simulink model "Sensors_Integrated"  (R2021b)
settings: Solver=FixedStepAuto  StartTime=0.0  StopTime=10.0  RelTol=1e-3
settings Model: Creator=Mohand  LastModifiedBy=Mohand
settings OptimizationCC: PassReuseOutputArgsAs=Individual arguments  OptimizeDataStoreBuffers=off  BusAssignmentInplaceUpdate=off  OptimizationLevel=level0  EfficientTunableParamExpr=on
settings DebuggingCC: ParameterTunabilityLossMsg=error
settings HardwareCC: ProdBitPerPointer=32  ProdBitPerSizeT=32  ProdBitPerPtrDiffT=32  ProdLargestAtomicInteger=Long  ProdLargestAtomicFloat=Double  ProdWordSize=32  ProdHWDeviceType=ARM Compatible->ARM Cortex-M
settings SFSimCC: MATLABDynamicMemAlloc=off
settings RTWCC: Description=Embedded Coder  SystemTargetFile=ert.tlc  GenCodeOnly=on  TemplateMakefile=ert_default_tmf  GenerateReport=on
settings CodeAppCC: ForceParamTrailComments=on  IgnoreCustomStorageClasses=off  OperatorAnnotations=on  SimulinkDataObjDesc=on  SFDataObjDesc=on  CustomSymbolStrGlobalVar=rt$N$M  CustomSymbolStrType=$N$M  CustomSymbolStrFcn=$N$M$F  InsertBlockDesc=on
settings ERTTargetCC: GenerateSampleERTMain=on  CodeInterfacePackaging=Reusable function  SupportComplex=off  SupportContinuousTime=on  ERTCustomFileTemplate=example_file_process.tlc

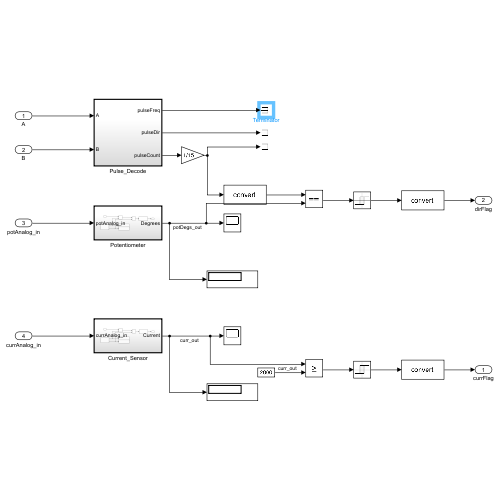
[thumbnail: Simulink's stored preview of the top-level diagram]
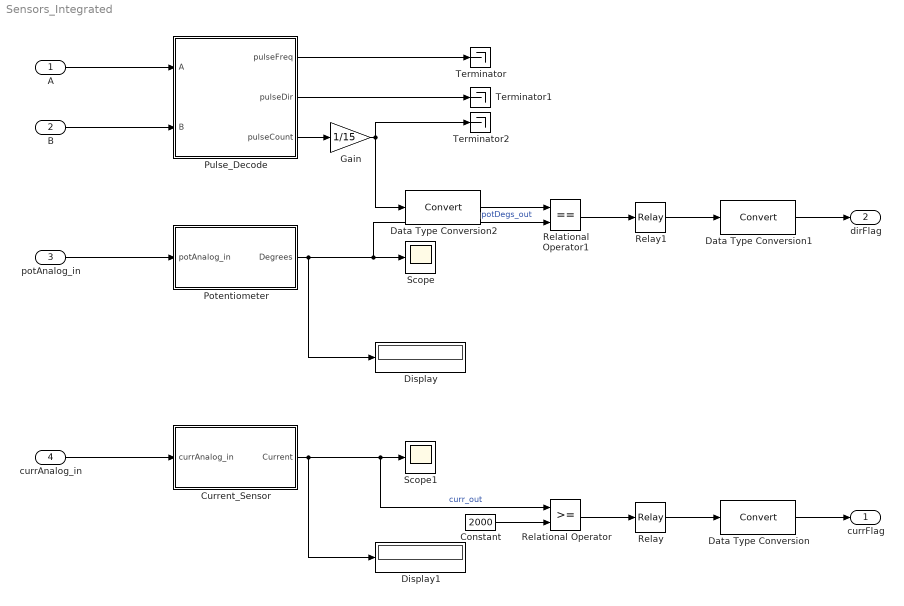
== system Sensors_Integrated ==
  A : Inport  OutDataTypeStr=uint8
  B : Inport  Port=2  OutDataTypeStr=uint8
  potAnalog_in : Inport  Port=3  OutDataTypeStr=uint8
  currAnalog_in : Inport  Port=4  OutDataTypeStr=uint8
  Constant : Constant  Value=2000  OutDataTypeStr=uint16
  Current_Sensor : Subsystem  TreatAsAtomicUnit=on
  Data Type Conversion : DataTypeConversion
  Data Type Conversion1 : DataTypeConversion
  Data Type Conversion2 : DataTypeConversion
  Display : Display
  Display1 : Display
  Gain : Gain  Gain=1/15
  Potentiometer : Subsystem  TreatAsAtomicUnit=on
  Pulse_Decode : Subsystem  TreatAsAtomicUnit=on
  Relational Operator : RelationalOperator  OutDataTypeStr=boolean  RndMeth=Simplest
  Relational Operator1 : RelationalOperator  Operator===  OutDataTypeStr=boolean  RndMeth=Simplest
  Relay : Relay  OnSwitchValue=1
  Relay1 : Relay  OnSwitchValue=1  OnOutputValue=0  OffOutputValue=1
  Scope : Scope
  Scope1 : Scope
  Terminator : Terminator
  Terminator1 : Terminator
  Terminator2 : Terminator
  currFlag : Outport  OutDataTypeStr=uint8
  dirFlag : Outport  Port=2  OutDataTypeStr=uint8
  wires:
  Potentiometer/1(Degrees) -> Relational Operator1/2, Scope/1, Display/1  "potDegs_out"
  potAnalog_in/1 -> Potentiometer/1(potAnalog_in)
  Current_Sensor/1(Current) -> Relational Operator/1, Scope1/1, Display1/1  "curr_out"
  currAnalog_in/1 -> Current_Sensor/1(currAnalog_in)
  B/1 -> Pulse_Decode/2(B)
  Pulse_Decode/2(pulseDir) -> Terminator1/1
  A/1 -> Pulse_Decode/1(A)
  Pulse_Decode/1(pulseFreq) -> Terminator/1
  Constant/1 -> Relational Operator/2
  Relational Operator/1 -> Relay/1
  Relay/1 -> Data Type Conversion/1
  Data Type Conversion/1 -> currFlag/1
  Data Type Conversion1/1 -> dirFlag/1
  Relay1/1 -> Data Type Conversion1/1
  Relational Operator1/1 -> Relay1/1
  Pulse_Decode/3(pulseCount) -> Gain/1
  Gain/1 -> Terminator2/1, Data Type Conversion2/1
  Data Type Conversion2/1 -> Relational Operator1/1

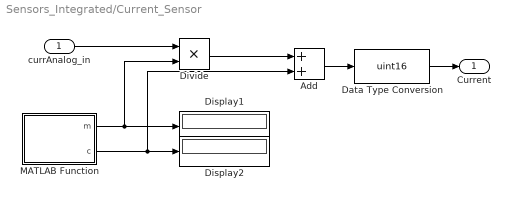
== system Sensors_Integrated/Current_Sensor ==
  currAnalog_in : Inport
  Add : Sum
  Data Type Conversion : DataTypeConversion  OutDataTypeStr=uint16
  Display1 : Display
  Display2 : Display
  Divide : Product  Inputs=**
  MATLAB Function : MATLAB Function  TreatAsAtomicUnit=on
  Current : Outport
  wires:
  currAnalog_in/1 -> Divide/1
  MATLAB Function/2(c) -> Add/2, Display2/1
  MATLAB Function/1(m) -> Divide/2, Display1/1
  Divide/1 -> Add/1
  Data Type Conversion/1 -> Current/1
  Add/1 -> Data Type Conversion/1

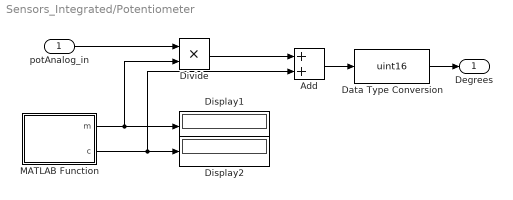
== system Sensors_Integrated/Potentiometer ==
  potAnalog_in : Inport
  Add : Sum
  Data Type Conversion : DataTypeConversion  OutDataTypeStr=uint16
  Display1 : Display
  Display2 : Display
  Divide : Product  Inputs=**
  MATLAB Function : MATLAB Function  TreatAsAtomicUnit=on
  Degrees : Outport
  wires:
  potAnalog_in/1 -> Divide/1
  MATLAB Function/2(c) -> Add/2, Display2/1
  MATLAB Function/1(m) -> Divide/2, Display1/1
  Divide/1 -> Add/1
  Data Type Conversion/1 -> Degrees/1
  Add/1 -> Data Type Conversion/1

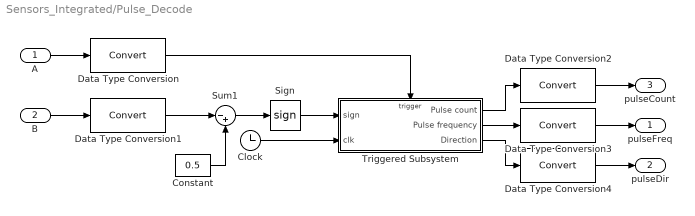
== system Sensors_Integrated/Pulse_Decode ==
  A : Inport
  B : Inport  Port=2
  Clock : Clock
  Constant : Constant  Value=0.5
  Data Type Conversion{,1..4} (5 alike) : DataTypeConversion
  Sign : Signum
  Sum1 : Sum  Inputs=|-+
  Triggered Subsystem : Subsystem  TreatAsAtomicUnit=on
  pulseFreq : Outport  VectorParamsAs1DForOutWhenUnconnected=off
  pulseDir : Outport  Port=2  VectorParamsAs1DForOutWhenUnconnected=off
  pulseCount : Outport  Port=3  VectorParamsAs1DForOutWhenUnconnected=off
  wires:
  Triggered Subsystem/3(Direction) -> Data Type Conversion4/1
  Triggered Subsystem/2(Pulse frequency) -> Data Type Conversion3/1
  Clock/1 -> Triggered Subsystem/2(clk)
  Triggered Subsystem/1(Pulse count) -> Data Type Conversion2/1
  A/1 -> Data Type Conversion/1
  Sign/1 -> Triggered Subsystem/1(sign)
  B/1 -> Data Type Conversion1/1
  Sum1/1 -> Sign/1
  Constant/1 -> Sum1/2
  Data Type Conversion/1 -> Triggered Subsystem/Trigger
  Data Type Conversion1/1 -> Sum1/1
  Data Type Conversion2/1 -> pulseCount/1
  Data Type Conversion3/1 -> pulseFreq/1
  Data Type Conversion4/1 -> pulseDir/1

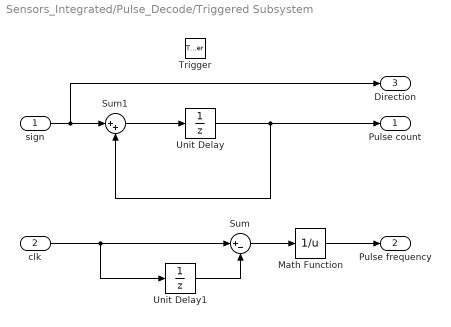
== system Sensors_Integrated/Pulse_Decode/Triggered Subsystem ==
  sign : Inport
  clk : Inport  Port=2
  Trigger : TriggerPort  VariantControl=Variant
  Math Function : Math  Operator=reciprocal  SignedPower=on  SaturateOnIntegerOverflow=on
  Sum : Sum  Inputs=|+-
  Sum1 : Sum  Inputs=|++
  Unit Delay : UnitDelay  SampleTime=-1  HasFrameUpgradeWarning=on
  Unit Delay1 : UnitDelay  InitialCondition=-1e10  SampleTime=-1  HasFrameUpgradeWarning=on
  Pulse count : Outport  InitialOutput=0  VectorParamsAs1DForOutWhenUnconnected=off
  Pulse frequency : Outport  Port=2  VectorParamsAs1DForOutWhenUnconnected=off
  Direction : Outport  Port=3  InitialOutput=0  VectorParamsAs1DForOutWhenUnconnected=off
  wires:
  Math Function/1 -> Pulse frequency/1
  Sum/1 -> Math Function/1
  Unit Delay1/1 -> Sum/2
  clk/1 -> Sum/1, Unit Delay1/1
  Unit Delay/1 -> Sum1/2, Pulse count/1
  sign/1 -> Direction/1, Sum1/1
  Sum1/1 -> Unit Delay/1

== matlab function Sensors_Integrated/Potentiometer/MATLAB Function ==
  data: m output; c output
function [m, c] = polyFcn_Pot()
x = [0     17      34      51     68     85     102     119     136     153     170     187     204     221     238     255];                 % Output in Bits
y = [0     24      48      72     96     120    144     168     192     216     240     264     288     312     336     360];                 % Angular Position in Degrees
n = 1;                                % Polynomial Order to Fit
p = polyfit(x,y,n);                   % Coeffs of fitted polynomial
m = p(1);
c = uint8(p(2));
% 
% x_fit = [0:1:300];
% y_fit = (p(1)*x_fit) + p(2);
% 
% plot(x_fit, y_fit, x, y, 'ro');
% xlabel('Output Voltage (Bits)');
% ylabel('Angular Position (Degrees)');
% legend('Fitted Curve', 'Recorded Data', 'Location', 'Northwest');

== matlab function Sensors_Integrated/Current_Sensor/MATLAB Function ==
  data: m output; c output
function [m, c] = polyFcn_Curr()
x = [0     17      34      51     68     85     102     119     136     153     170     187     204     221     238     255];                 % Output in Bits
y = [0     10      20      30     40     50     60      70      80      90      100     110     120     130     140     150];                 % Current in mA
n = 1;                                % Polynomial Order to Fit
p = polyfit(x,y,n);                   % Coeffs of fitted polynomial
m = p(1);
c = uint8(p(2));
% 
% x_fit = [0:1:300];
% y_fit = (p(1)*x_fit) + p(2);
% 
% plot(x_fit, y_fit, x, y, 'ro');
% xlabel('Output Voltage (Bits)');
% ylabel('Angular Position (Degrees)');
% legend('Fitted Curve', 'Recorded Data', 'Location', 'Northwest');
